simulink library "PE3PHABLO01MSEREF"  (R2014b)
settings: Solver=ode45  StartTime=0.0  StopTime=10.0  RelTol=1e-3
libraries: PE3PHABLO01MSEREF x2
settings Model: Creator=vda2sh  LastModifiedBy=vda2sh

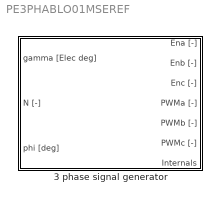
== system PE3PHABLO01MSEREF ==
  3 phase signal generator : Subsystem  Tag=PE3PHABLO01MSEREF  mask(PE3PHABLO01MSEREF){beta=120, range=0 to 1}
      mask prompts: beta "Block width [Elec deg]"; range "PWM range"
      mask help:
      | PE3PHABLO01MSEREF - 3 phase signal generator
      |
      | This block generates signals to command the drive (i.e., the B6-bridge) of an electric powertrain.
      settings: AttributesFormatString=<%<Tag>>
      mask Help: eval('show_docs_mseref_powerelectronics(''PE3PHABLO01MSEREF'')')
      mask TypeOptions range: 0 to 1 | -1 to 1
      mask Display:
      | image(imread('PE3PHABLO01MSEREF.png'),[0.02,0.12, 0.8,0.7]);
      | port_label('input', 1, 'gamma [Elec deg]');
      | port_label('input', 2, 'N [-]');
      | port_label('input', 3, 'phi [deg]');
      | port_label('output', 1, 'Ena [-]');
      | port_label('output', 2, 'Enb [-]');
      | port_label('output', 3, 'Enc [-]');
      | port_label('output', 4, 'PWMa [-]');
      | port_label('output', 5, 'PWMb [-]');
      | port_label('output', 6, 'PWMc [-]');
      | port_label('output', 7, 'Internals');

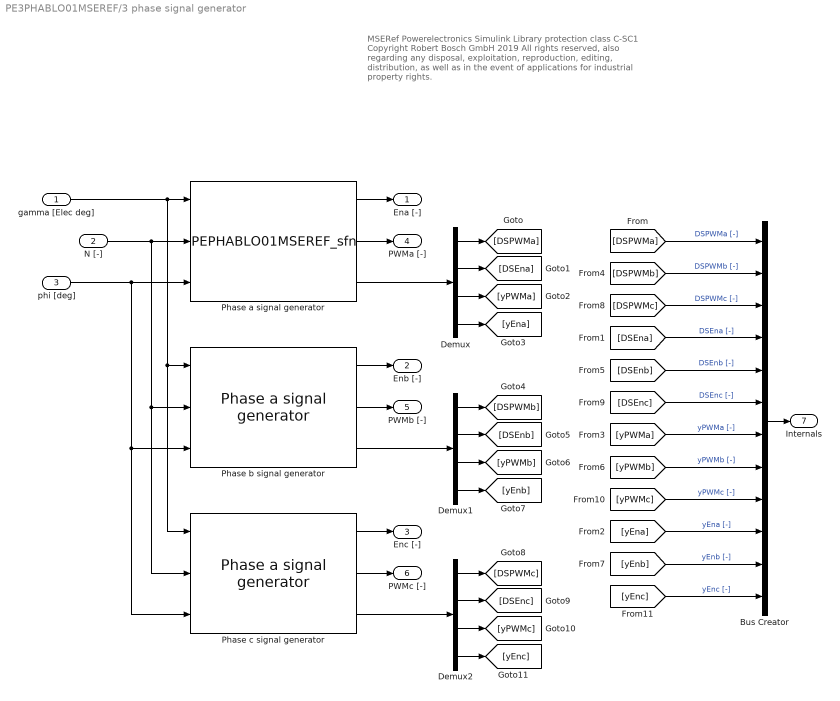
== system PE3PHABLO01MSEREF/3 phase signal generator ==
  note: MSERef Powerelectronics Simulink Library
      | protection class C-SC1
      |
      | Copyright Robert Bosch GmbH 2019
      |
      | All rights reserved, also regarding any disposal, exploitation,
      | reproduction, editing, distribution, as well as in the event of
      | applications for industrial property rights.
  gamma [Elec deg] : Inport
  N [-] : Inport  Port=2
  phi [deg] : Inport  Port=3
  Bus Creator : BusCreator  Inputs=12
  Demux : Demux
  Demux1 : Demux
  Demux2 : Demux
  Phase a signal generator : S-Function  Tag=PEPHABLO01MSEREF  FunctionName=PEPHABLO01MSEREF_sfn  Parameters=beta, range, phi_offset  EnableBusSupport=off  mask{beta=beta, range=range, phi_offset=0}
      mask prompts: beta "Block width [Elec deg]"; range "PWM range [-]"; phi_offset "Offset angle [Elec deg]"
      settings: AttributesFormatString=<%<Tag>>
      mask Display:
      | port_label('input', 1, 'gamma [Elec deg]');
      | port_label('input', 2, 'N [-]');
      | port_label('input', 3, 'phi [deg]');
      | port_label('output', 1, 'En [-]');
      | port_label('output', 2, 'PWM [-]');
      | port_label('output', 3, 'Internals');
  Phase b signal generator : PE3PHABLO01MSEREF/3 phase signal generator/Phase a signal generator  Tag=PEPHABLO01MSEREF  beta=beta  range=range  phi_offset=120
      settings: AttributesFormatString=<%<Tag>>
  Phase c signal generator : PE3PHABLO01MSEREF/3 phase signal generator/Phase a signal generator  Tag=PEPHABLO01MSEREF  beta=beta  range=range  phi_offset=240
      settings: AttributesFormatString=<%<Tag>>
  Ena [-] : Outport
  Enb [-] : Outport  Port=2
  Enc [-] : Outport  Port=3
  PWMa [-] : Outport  Port=4
  PWMb [-] : Outport  Port=5
  PWMc [-] : Outport  Port=6
  Internals : Outport  Port=7
  wires:
  gamma [Elec deg]/1 -> Phase c signal generator/1, Phase b signal generator/1, Phase a signal generator/1
  N [-]/1 -> Phase c signal generator/2, Phase b signal generator/2, Phase a signal generator/2
  phi [deg]/1 -> Phase c signal generator/3, Phase b signal generator/3, Phase a signal generator/3
  Phase a signal generator/1 -> Ena [-]/1
  Phase a signal generator/2 -> PWMa [-]/1
  Phase b signal generator/1 -> Enb [-]/1
  Phase c signal generator/1 -> Enc [-]/1
  Phase b signal generator/2 -> PWMb [-]/1
  Phase c signal generator/2 -> PWMc [-]/1
  Bus Creator/1 -> Internals/1
  Demux/1 -> [DSPWMa]
  Phase a signal generator/3 -> Demux/1
  Demux/2 -> [DSEna]
  Demux/3 -> [yPWMa]
  Demux/4 -> [yEna]
  Demux1/1 -> [DSPWMb]
  Phase b signal generator/3 -> Demux1/1
  Demux1/2 -> [DSEnb]
  Demux1/3 -> [yPWMb]
  Demux1/4 -> [yEnb]
  Demux2/1 -> [DSPWMc]
  Demux2/2 -> [DSEnc]
  Demux2/3 -> [yPWMc]
  Demux2/4 -> [yEnc]
  Phase c signal generator/3 -> Demux2/1
  [DSPWMa] -> Bus Creator/1  "DSPWMa [-]"
  [DSEna] -> Bus Creator/4  "DSEna [-]"
  [yEna] -> Bus Creator/10  "yEna [-]"
  [yPWMa] -> Bus Creator/7  "yPWMa [-]"
  [DSPWMb] -> Bus Creator/2  "DSPWMb [-]"
  [DSEnb] -> Bus Creator/5  "DSEnb [-]"
  [yPWMb] -> Bus Creator/8  "yPWMb [-]"
  [yEnb] -> Bus Creator/11  "yEnb [-]"
  [DSPWMc] -> Bus Creator/3  "DSPWMc [-]"
  [DSEnc] -> Bus Creator/6  "DSEnc [-]"
  [yPWMc] -> Bus Creator/9  "yPWMc [-]"
  [yEnc] -> Bus Creator/12  "yEnc [-]"
